simulink library "Valeo_Simulink_Library_EC"  (R2017b)
settings: Solver=ode45  StartTime=0.0  StopTime=10.0  RelTol=1e-3  EnableMultiTasking=on
undefined symbols (not defined in the file): A, B, C, Count_Max, D, InitValue, j, ke, kf, kt, L, Length, MaxIniVal, MaxVal, MinVal, NumBits1, NumBits2, P, p0, Q, R, Simulink_Library, Ts, x0
libraries: Valeo_Simulink_Library_EC x9, simulink x8, fixpt_dtprop x4
(part 3 of 3)

== system Valeo_Simulink_Library_EC/Signal_Operations/TurnOffDelay ==
  In : Inport
  Tdly : Inport  Port=2
  Te : Inport  Port=3
  CheckDly : RelationalOperator  Operator=<  OutDataTypeStr=boolean  RndMeth=Nearest  InputSameDT=on
  Check_Tdly_unsigned : fixpt_dtprop/Data Type Police Unsigned Only
      settings: SourceProductName=Simulink  SourceProductBaseCode=SL
  Check_Te_unsigned : fixpt_dtprop/Data Type Police Unsigned Only
      settings: SourceProductName=Simulink  SourceProductBaseCode=SL
  Divide : Product  Inputs=*/  OutDataTypeStr=uint32  RndMeth=Nearest  SaturateOnIntegerOverflow=on
  Inc : Constant  OutDataTypeStr=Inherit: Inherit via back propagation
  Increment : Sum  OutDataTypeStr=Inherit: Inherit via back propagation  SaturateOnIntegerOverflow=on  InputSameDT=on
  InitialCondition : Subsystem  Description=InitialCondition
  LogicalOperator : Logic  Operator=OR  AllPortsSameDT=off  OutDataTypeStr=boolean
  NewVal : UnitDelay  SampleTime=-1
  Reset : Constant  Value=0  OutDataTypeStr=Inherit: Inherit via back propagation
  ResetSwitch : Switch  Criteria=u2 ~= 0  InputSameDT=on
  StartDelay : UnitDelay  SampleTime=-1
  Out : Outport
  wires:
  LogicalOperator/1 -> Out/1
  Reset/1 -> ResetSwitch/1
  ResetSwitch/1 -> Increment/1, CheckDly/1
  Increment/1 -> NewVal/1
  CheckDly/1 -> LogicalOperator/1
  In/1 -> LogicalOperator/2, InitialCondition/1(CheckDir), StartDelay/1
  NewVal/1 -> InitialCondition/3(NewVal)
  InitialCondition/1(CalcVal) -> ResetSwitch/3
  StartDelay/1 -> ResetSwitch/2
  Divide/1 -> CheckDly/2, InitialCondition/2(Tdly)
  Te/1 -> Check_Te_unsigned/1, Divide/2
  Tdly/1 -> Check_Tdly_unsigned/1, Divide/1
  Inc/1 -> Increment/2

== system Valeo_Simulink_Library_EC/Signal_Operations/TurnOnDelay ==
  In : Inport
  Tdly : Inport  Port=2
  Te : Inport  Port=3
  CheckDly : RelationalOperator  OutDataTypeStr=boolean  RndMeth=Nearest  InputSameDT=on
  Check_Tdly_unsigned : fixpt_dtprop/Data Type Police Unsigned Only
      settings: SourceProductName=Simulink  SourceProductBaseCode=SL
  Check_Te_unsigned : fixpt_dtprop/Data Type Police Unsigned Only
      settings: SourceProductName=Simulink  SourceProductBaseCode=SL
  Divide : Product  Inputs=*/  OutDataTypeStr=uint32  SaturateOnIntegerOverflow=on
  Inc : Constant  OutDataTypeStr=Inherit: Inherit via back propagation
  Increment : Sum  OutDataTypeStr=Inherit: Inherit via back propagation  RndMeth=Simplest  SaturateOnIntegerOverflow=on  InputSameDT=on
  InitialCondition : Subsystem  Description=InitialCondition
  InitialDelayl : UnitDelay  InitialCondition=1  SampleTime=-1
  LogicalOperator : Logic  AllPortsSameDT=off  OutDataTypeStr=boolean
  NewVal : UnitDelay  SampleTime=-1
  Reset : Constant  Value=0  OutDataTypeStr=Inherit: Inherit via back propagation
  ResetSwitch : Switch  Criteria=u2 ~= 0  InputSameDT=on
  Out : Outport
  wires:
  InitialDelayl/1 -> ResetSwitch/2
  LogicalOperator/1 -> Out/1
  ResetSwitch/1 -> Increment/1, CheckDly/1
  Increment/1 -> NewVal/1
  CheckDly/1 -> LogicalOperator/1
  NewVal/1 -> InitialCondition/1(NewVal)
  In/1 -> LogicalOperator/2, InitialCondition/3(CheckDir), InitialDelayl/1
  InitialCondition/1(CalcVal) -> ResetSwitch/1
  Reset/1 -> ResetSwitch/3
  Tdly/1 -> Divide/1, Check_Tdly_unsigned/1
  Te/1 -> Divide/2, Check_Te_unsigned/1
  Divide/1 -> InitialCondition/2(Tdly), CheckDly/2
  Inc/1 -> Increment/2

== system Valeo_Simulink_Library_EC/Signal_Operations/VSL_ClarkTransformation_EC_Blk ==
  A : Inport  PortDimensions=1
  B : Inport  Port=2  PortDimensions=1
  C : Inport  Port=3  PortDimensions=1
  Calculation : Subsystem  Description=Calculations for clarke transfromation  RequirementInfo={} %GIDa_91c9902b_4297_47d8_bcc7_839692c95106
  datatype_protection : Subsystem  Description=forcing input and output to have the same data type  RequirementInfo={} %GIDa_ba0677aa_132e_4dc0_8af7_6cee4e109de7
  Alpha : Outport  RequirementInfo={} %GIDa_2f11082c_73d3_4ed4_8929_d03a8ab0ed51  PortDimensions=1
  Beta : Outport  RequirementInfo={} %GIDa_b2cc2919_a1d0_479c_944a_1162b348937b  Port=2  PortDimensions=1
  wires:
  [C] -> datatype_protection/5(C)
  [B] -> datatype_protection/4(B)
  [A] -> datatype_protection/3(A)
  Calculation/2(Beta) -> datatype_protection/2(Beta_temp)
  Calculation/1(Alpha) -> datatype_protection/1(Alpha_temp)
  datatype_protection/2(Beta) -> Beta/1
  datatype_protection/1(Alpha) -> Alpha/1
  [C] -> Calculation/3(C)
  [B] -> Calculation/2(B)
  [A] -> Calculation/1(A)
  C/1 -> [C]  "C"
  A/1 -> [A]  "A"
  B/1 -> [B]  "B"

== system Valeo_Simulink_Library_EC/Signal_Operations/VSL_InverseClarkTransformation_EC_Blk ==
  Alpha : Inport
  Beta : Inport  Port=2
  Calculations : Subsystem  Description=claclulations of Inverse clarke transform
  "DataTypeProtection " : Subsystem  Description=make sure all inputs and outputs have the same datatype
  A : Outport
  B : Outport  Port=2
  C : Outport  Port=3
  wires:
  Beta/1 -> [Beta]
  Alpha/1 -> [Alpha]
  [Beta] -> "DataTypeProtection "/5(Beta)
  [Alpha] -> "DataTypeProtection "/4(Alpha)
  [Beta] -> Calculations/2(Beta)
  [Alpha] -> Calculations/1(Alpha)
  "DataTypeProtection "/3(C) -> C/1
  "DataTypeProtection "/2(B) -> B/1
  "DataTypeProtection "/1(A) -> A/1
  Calculations/3(C) -> "DataTypeProtection "/3(C_t)
  Calculations/2(B) -> "DataTypeProtection "/2(B_t)
  Calculations/1(A) -> "DataTypeProtection "/1(A_t)

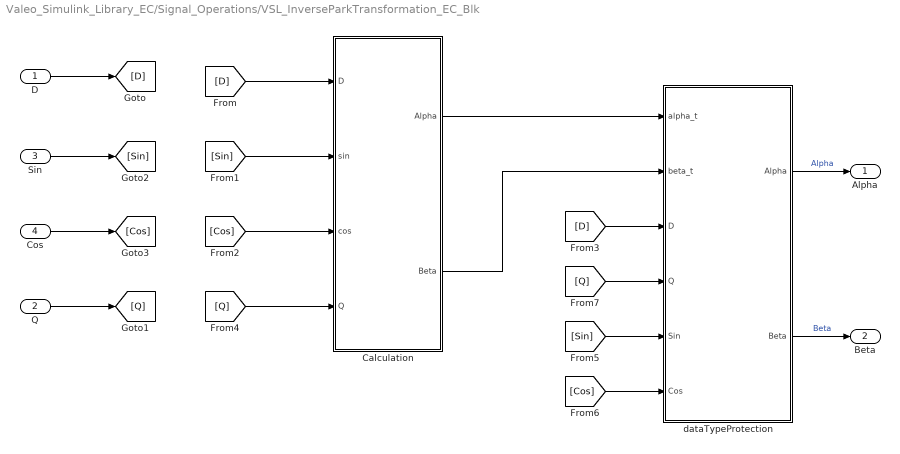
== system Valeo_Simulink_Library_EC/Signal_Operations/VSL_InverseParkTransformation_EC_Blk ==
  D : Inport
  Q : Inport  Port=2
  Sin : Inport  Port=3
  Cos : Inport  Port=4
  Calculation : Subsystem  Description=This Block is transforming dq axies with d axis aligned with Phase A into alpha-beta axises
      settings: RTWFcnNameOpts=Use subsystem name
  dataTypeProtection : Subsystem  Description=make sure inputs and outputs have the same data type
  Alpha : Outport
  Beta : Outport  Port=2
  wires:
  Calculation/1(Alpha) -> dataTypeProtection/1(alpha_t)
  Calculation/2(Beta) -> dataTypeProtection/2(beta_t)
  Q/1 -> [Q]
  D/1 -> [D]
  [D] -> Calculation/1(D)
  [Q] -> Calculation/4(Q)
  Sin/1 -> [Sin]
  Cos/1 -> [Cos]
  [Sin] -> Calculation/2(sin)
  [Cos] -> Calculation/3(cos)
  dataTypeProtection/2(Beta) -> Beta/1  "Beta"
  dataTypeProtection/1(Alpha) -> Alpha/1  "Alpha"
  [D] -> dataTypeProtection/3(D)
  [Q] -> dataTypeProtection/4(Q)
  [Sin] -> dataTypeProtection/5(Sin)
  [Cos] -> dataTypeProtection/6(Cos)

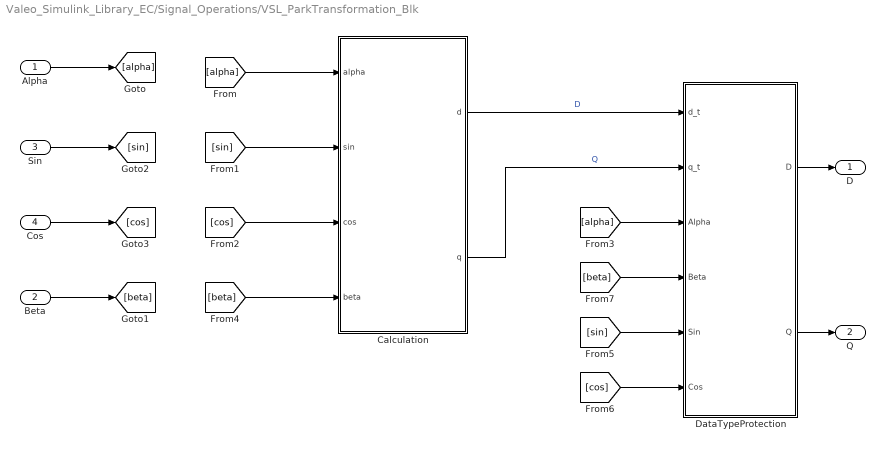
== system Valeo_Simulink_Library_EC/Signal_Operations/VSL_ParkTransformation_Blk ==
  Alpha : Inport
  Beta : Inport  Port=2
  Sin : Inport  Port=3
  Cos : Inport  Port=4
  Calculation : Subsystem  Description=This Block is transforming alpha-beta axises into dq axies with d axie aligned with Phase A
      settings: RTWSystemCode=Nonreusable function  RTWFcnNameOpts=Use subsystem name
  DataTypeProtection : Subsystem  Description=make sure all inputs and outputs have the sane data type
  D : Outport
  Q : Outport  Port=2
  wires:
  [cos] -> DataTypeProtection/6(Cos)
  [sin] -> DataTypeProtection/5(Sin)
  [beta] -> DataTypeProtection/4(Beta)
  [alpha] -> DataTypeProtection/3(Alpha)
  DataTypeProtection/2(Q) -> Q/1
  DataTypeProtection/1(D) -> D/1
  [cos] -> Calculation/3(cos)
  [sin] -> Calculation/2(sin)
  Cos/1 -> [cos]
  Sin/1 -> [sin]
  Calculation/2(q) -> DataTypeProtection/2(q_t)  "Q"
  Calculation/1(d) -> DataTypeProtection/1(d_t)  "D"
  [beta] -> Calculation/4(beta)
  [alpha] -> Calculation/1(alpha)
  Alpha/1 -> [alpha]
  Beta/1 -> [beta]

== system Valeo_Simulink_Library_EC/Utilities/EventToVar ==
  Evt : Inport
  Constant1 : Constant  Value=0  OutDataTypeStr=boolean  SampleTime=-1
  Constant2 : Constant  OutDataTypeStr=boolean  SampleTime=-1
  Function-Call Subsystem : Subsystem  Description=|  TreatAsAtomicUnit=on
      | Function-Call
      | Subsystem
  Logical Operator1 : Logic  Tag=AM,Std,Inputs,1;CMP,Operator,Inputs;  Operator=NOT  Inputs=1  AllPortsSameDT=off  OutDataTypeStr=boolean
  Relational Operator : RelationalOperator  Operator=~=  OutDataTypeStr=boolean  RndMeth=Nearest
  Switch : Switch  Criteria=u2 ~= 0
  Unit Delay1 : UnitDelay  SampleTime=-1
  Unit Delay2 : UnitDelay  SampleTime=-1
  Var : Outport
  wires:
  Logical Operator1/1 -> Relational Operator/1, Unit Delay1/1
  Switch/1 -> Var/1
  Relational Operator/1 -> Switch/2
  Constant1/1 -> Switch/3
  Constant2/1 -> Switch/1
  Unit Delay1/1 -> Relational Operator/2
  Function-Call Subsystem/1(out) -> Logical Operator1/1, Unit Delay2/1
  Unit Delay2/1 -> Function-Call Subsystem/1(in)
  Evt/1 -> Function-Call Subsystem/Trigger

== system Valeo_Simulink_Library_EC/Utilities/ScribeInfo ==

== system Valeo_Simulink_Library_EC/Plant Models/Actuators/BLDC ==
  Vs : Inport
  TL : Inport  Port=2
  BLDC motor Block : Subsystem
  inverter : Subsystem
  Te : Outport
  omega(rad/sec) : Outport  Port=2
  Position : Outport  Port=3
  i_abc : Outport  Port=4
  wires:
  BLDC motor Block/4(B_EMF) -> inverter/3(B_EMF)
  BLDC motor Block/1(Te) -> Te/1
  BLDC motor Block/3(Position) -> Position/1, inverter/1(POS)
  inverter/1("Uab, Ubc") -> BLDC motor Block/1(" Uab,Ubc")
  TL/1 -> BLDC motor Block/2(Tl)
  BLDC motor Block/5(i_abc) -> inverter/4(i_abc), i_abc/1
  Vs/1 -> inverter/2(Vs)
  BLDC motor Block/2(Omega) -> omega(rad/sec)/1  "omega(rad/sec)"

== system Valeo_Simulink_Library_EC/Signal_Operations/Debouncing_Blk/Else ==
  In : Inport
  Action Port : ActionPort
  Signal Conversion : SignalConversion  OverrideOpt=off
  Out : Outport
  wires:
  In/1 -> Signal Conversion/1
  Signal Conversion/1 -> Out/1

== system Valeo_Simulink_Library_EC/Signal_Operations/Debouncing_Blk/Turn_OFF ==
  Action Port : ActionPort
  Constant1 : Constant  Value=0  OutDataTypeStr=uint8  SampleTime=-1
  Constant3 : Constant  Value=0  OutDataTypeStr=boolean  SampleTime=-1
  Counter : Outport
  Out : Outport  Port=2
  wires:
  Constant3/1 -> Out/1
  Constant1/1 -> Counter/1

== system Valeo_Simulink_Library_EC/Signal_Operations/Debouncing_Blk/Turn_ON ==
  Action Port : ActionPort
  Constant3 : Constant  Value=0  OutDataTypeStr=uint8  SampleTime=-1
  Constant4 : Constant  OutDataTypeStr=boolean  SampleTime=-1
  Out : Outport
  Counter : Outport  Port=2
  wires:
  Constant4/1 -> Out/1
  Constant3/1 -> Counter/1

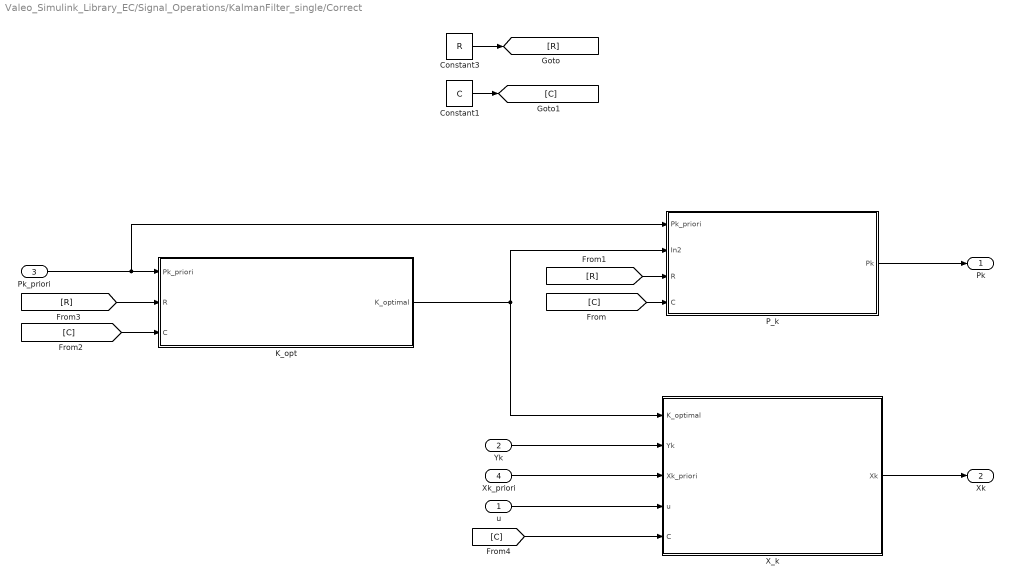
== system Valeo_Simulink_Library_EC/Signal_Operations/KalmanFilter_single/Correct ==
  u : Inport
  Yk : Inport  Port=2
  Pk_priori : Inport  Port=3
  Xk_priori : Inport  Port=4
  Constant1 : Constant  Value=C  VectorParams1D=off  OutDataTypeStr=single
  Constant3 : Constant  Value=R  VectorParams1D=off  OutDataTypeStr=single
  K_opt : Subsystem
  P_k : Subsystem
  X_k : Subsystem
  Pk : Outport  OutDataTypeStr=single  InitialOutput=0
  Xk : Outport  Port=2  OutDataTypeStr=single  InitialOutput=3
  wires:
  Pk_priori/1 -> P_k/1(Pk_priori), K_opt/1(Pk_priori)
  Constant3/1 -> [R]
  Yk/1 -> X_k/2(Yk)
  Xk_priori/1 -> X_k/3(Xk_priori)
  u/1 -> X_k/4(u)
  X_k/1(Xk) -> Xk/1
  Constant1/1 -> [C]
  [C] -> X_k/5(C)
  K_opt/1(K_optimal) -> X_k/1(K_optimal), P_k/2(In2)
  P_k/1(Pk) -> Pk/1
  [R] -> P_k/3(R)
  [C] -> P_k/4(C)
  [R] -> K_opt/2(R)
  [C] -> K_opt/3(C)

== system Valeo_Simulink_Library_EC/Signal_Operations/KalmanFilter_single/Predict ==
  u : Inport
  Pk-1 : Inport  Port=2
  Xk-1 : Inport  Port=3
  Add : Sum
  Add1 : Sum
  Constant : Constant  Value=A  VectorParams1D=off  OutDataTypeStr=single
  Constant1 : Constant  Value=Q  VectorParams1D=off  OutDataTypeStr=single
  Constant2 : Constant  Value=B  VectorParams1D=off  OutDataTypeStr=single
  Math Function : Math  Operator=transpose  SaturateOnIntegerOverflow=on
  Product : Product  Inputs=3  Multiplication=Matrix(*)
  Product1 : Product  Inputs=**  Multiplication=Matrix(*)  RndMeth=Zero
  Product2 : Product  Inputs=**  Multiplication=Matrix(*)  RndMeth=Zero
  Pk_priori : Outport  OutDataTypeStr=single
  Xk_priori : Outport  Port=2  OutDataTypeStr=single
  wires:
  Constant2/1 -> Product2/1
  Math Function/1 -> Product/3
  Constant/1 -> Product/1, Product1/1, Math Function/1
  Product/1 -> Add1/2
  Pk-1/1 -> Product/2
  Product1/1 -> Add/1
  Xk-1/1 -> Product1/2
  u/1 -> Product2/2
  Product2/1 -> Add/2
  Add1/1 -> Pk_priori/1
  Constant1/1 -> Add1/1
  Add/1 -> Xk_priori/1

== system Valeo_Simulink_Library_EC/Signal_Operations/NegHys/Hysteresis ==
  Low : Inport
  In : Inport  Port=2
  High : Inport  Port=3
  RemainderIN : Inport  Port=4
  Constant : Constant  Value=0  OutDataTypeStr=boolean
  Constant1 : Constant  OutDataTypeStr=boolean
  RelationalOperator3 : RelationalOperator  OutDataTypeStr=boolean  RndMeth=Nearest  InputSameDT=on
  RelationalOperator4 : RelationalOperator  OutDataTypeStr=boolean  RndMeth=Nearest  InputSameDT=on
  Switch : Switch  Criteria=u2 ~= 0  OutDataTypeStr=Inherit: Inherit via back propagation  InputSameDT=on
  Switch1 : Switch  Criteria=u2 ~= 0  OutDataTypeStr=Inherit: Inherit via back propagation  InputSameDT=on
  Out : Outport
  wires:
  RemainderIN/1 -> Switch1/3
  Switch/1 -> Out/1
  Switch1/1 -> Switch/3
  RelationalOperator4/1 -> Switch1/2
  Constant/1 -> Switch1/1
  RelationalOperator3/1 -> Switch/2
  Constant1/1 -> Switch/1
  Low/1 -> RelationalOperator3/1
  High/1 -> RelationalOperator4/2
  In/1 -> RelationalOperator4/1, RelationalOperator3/2

== system Valeo_Simulink_Library_EC/Signal_Operations/PosHys/Hysteresis ==
  Low : Inport
  In : Inport  Port=2
  High : Inport  Port=3
  RemainderIN : Inport  Port=4
  Constant : Constant  OutDataTypeStr=boolean
  Constant1 : Constant  Value=0  OutDataTypeStr=boolean
  RelationalOperator3 : RelationalOperator  OutDataTypeStr=boolean  RndMeth=Nearest  InputSameDT=on
  RelationalOperator4 : RelationalOperator  OutDataTypeStr=boolean  RndMeth=Nearest  InputSameDT=on
  Switch : Switch  Criteria=u2 ~= 0  OutDataTypeStr=Inherit: Inherit via back propagation  InputSameDT=on
  Switch1 : Switch  Criteria=u2 ~= 0  OutDataTypeStr=Inherit: Inherit via back propagation  InputSameDT=on
  Out : Outport
  wires:
  In/1 -> RelationalOperator3/2, RelationalOperator4/1
  High/1 -> RelationalOperator4/2
  Low/1 -> RelationalOperator3/1
  Constant1/1 -> Switch/1
  RelationalOperator3/1 -> Switch/2
  Constant/1 -> Switch1/1
  RelationalOperator4/1 -> Switch1/2
  Switch1/1 -> Switch/3
  Switch/1 -> Out/1
  RemainderIN/1 -> Switch1/3

== system Valeo_Simulink_Library_EC/Signal_Operations/SlidingAverageFiltrer/DPropagation_32Bits ==
  Ref1 : Inport
  DataProp : Inport  Port=2
  Data Type Propagation : simulink/Signal Attributes/Data Type Propagation  PropDataType=fixdt(1, 16)  IfRefDouble=double  IfRefSingle=single  IsSigned=TRUE  NumBitsBase=NumBits1  NumBitsMult=1  NumBitsAdd=0  NumBitsAllowFinal=8:32  PropScaling=2^-10  ValuesUsedBestPrec=[5 -7]  SlopeBase=Slope1  SlopeMult=1  SlopeAdd=0  BiasBase=Bias1  BiasMult=1  BiasAdd=0
      settings: SourceProductName=Simulink  SourceProductBaseCode=SL
  wires:
  Ref1/1 -> Data Type Propagation/2, Data Type Propagation/1
  DataProp/1 -> Data Type Propagation/3

== system Valeo_Simulink_Library_EC/Signal_Operations/SlidingAverageFiltrer/DPropagation_Others ==
  Ref1 : Inport
  DataProp : Inport  Port=2
  Data Type Propagation : simulink/Signal Attributes/Data Type Propagation  PropDataType=fixdt(1, 16)  IfRefDouble=double  IfRefSingle=single  IsSigned=TRUE  NumBitsBase=NumBits1+NumBits2  NumBitsMult=1  NumBitsAdd=0  NumBitsAllowFinal=8:32  PropScaling=2^-10  ValuesUsedBestPrec=[5 -7]  SlopeBase=Slope1  SlopeMult=1  SlopeAdd=0  BiasBase=Bias1  BiasMult=1  BiasAdd=0
      settings: SourceProductName=Simulink  SourceProductBaseCode=SL
  wires:
  DataProp/1 -> Data Type Propagation/3
  Ref1/1 -> Data Type Propagation/2, Data Type Propagation/1

== system Valeo_Simulink_Library_EC/Signal_Operations/SlidingAverageFiltrer/DPropagation_WindowLength ==
  Ref1 : Inport
  Ref2 : Inport  Port=2
  Prop : Inport  Port=3
  Data Type Propagation : simulink/Signal Attributes/Data Type Propagation  PropDataType=fixdt(1, 16)  IfRefDouble=double  IfRefSingle=single  IsSigned=FALSE  NumBitsBase=NumBits1  NumBitsMult=1  NumBitsAdd=0  NumBitsAllowFinal=8:32  PropScaling=2^-10  ValuesUsedBestPrec=[5 -7]  SlopeBase=Slope1  SlopeMult=1  SlopeAdd=0  BiasBase=Bias1  BiasMult=1  BiasAdd=0
      settings: SourceProductName=Simulink  SourceProductBaseCode=SL
  wires:
  Ref1/1 -> Data Type Propagation/1
  Ref2/1 -> Data Type Propagation/2
  Prop/1 -> Data Type Propagation/3

== system Valeo_Simulink_Library_EC/Signal_Operations/TurnOffDelay/InitialCondition ==
  CheckDir : Inport
  Tdly : Inport  Port=2
  NewVal : Inport  Port=3
  LogicalOperator1 : Logic  Operator=OR  AllPortsSameDT=off  OutDataTypeStr=boolean
  NewVal1 : UnitDelay  InitialCondition=1  SampleTime=-1
  Reset : Constant  Value=0  OutDataTypeStr=boolean
  Switch : Switch  Criteria=u2 ~= 0  InputSameDT=on
  CalcVal : Outport
  wires:
  NewVal/1 -> Switch/3
  Tdly/1 -> Switch/1
  NewVal1/1 -> LogicalOperator1/2
  Reset/1 -> NewVal1/1
  LogicalOperator1/1 -> Switch/2
  CheckDir/1 -> LogicalOperator1/1
  Switch/1 -> CalcVal/1

== system Valeo_Simulink_Library_EC/Signal_Operations/TurnOnDelay/InitialCondition ==
  NewVal : Inport
  Tdly : Inport  Port=2
  CheckDir : Inport  Port=3
  LogicalOperator : Logic  Operator=NOT  AllPortsSameDT=off  OutDataTypeStr=boolean
  LogicalOperator1 : Logic  Operator=OR  AllPortsSameDT=off  OutDataTypeStr=boolean
  NewVal1 : UnitDelay  SampleTime=-1
  Reset : Constant  OutDataTypeStr=boolean
  Switch : Switch  Criteria=u2 ~= 0  InputSameDT=on
  CalcVal : Outport
  wires:
  NewVal/1 -> Switch/1
  NewVal1/1 -> LogicalOperator1/2
  Reset/1 -> NewVal1/1
  LogicalOperator1/1 -> Switch/2
  Switch/1 -> CalcVal/1
  Tdly/1 -> Switch/3
  CheckDir/1 -> LogicalOperator/1
  LogicalOperator/1 -> LogicalOperator1/1

== system Valeo_Simulink_Library_EC/Signal_Operations/VSL_ClarkTransformation_EC_Blk/Calculation ==
  A : Inport
  B : Inport  Port=2
  C : Inport  Port=3
  Add : Sum  RequirementInfo={} %GIDa_afe2c577_734f_4faf_b375_0ef20aeeab01  Inputs=+++  OutDataTypeStr=Inherit: Inherit via back propagation  RndMeth=Simplest
  Add1 : Sum  RequirementInfo={} %GIDa_b8b12de4_a1c3_404a_a9d1_be098477dac5  OutDataTypeStr=Inherit: Inherit via back propagation  RndMeth=Simplest
  Const_2Over3 : Gain  Description=gain of 0.666 as 0.666  RequirementInfo={} %GIDa_120f91ab_5e07_4588_9a66_f8fa17d7ebbb  Gain=0.6667  OutDataTypeStr=Inherit: Inherit via back propagation  RndMeth=Simplest  ParamDataTypeStr=Inherit: Same as input
  Const_Neg1Over3 : Gain  Description=gain of -.333 as -.333  RequirementInfo={} %GIDa_cbff4a56_eba5_4d1b_82e9_2b912c46c30a  Gain=-.3333  OutDataTypeStr=Inherit: Inherit via back propagation  RndMeth=Simplest  ParamDataTypeStr=Inherit: Same as input
  Const_Neg1Over3_2 : Gain  Description=gain of -.333 as -.333  RequirementInfo={} %GIDa_82831831_6244_46f4_8700_983a6e4d662e  Gain=-.3333  OutDataTypeStr=Inherit: Inherit via back propagation  RndMeth=Simplest  ParamDataTypeStr=Inherit: Same as input
  Const_NegSqrt3Over3 : Gain  Description=gain of -.577 as -sqrt(3)/3  RequirementInfo={} %GIDa_a4218fb9_5262_4d86_8cc2_5cb31cf1db53  Gain=-.5773  OutDataTypeStr=Inherit: Inherit via back propagation  RndMeth=Simplest  ParamDataTypeStr=Inherit: Same as input
  Const_Sqrt3Over2 : Gain  Description=gain of .577 as sqrt(3)/3  RequirementInfo={} %GIDa_f78375a3_f7cc_4d79_b4c2_30115ac82f8c  Gain=.5773  OutDataTypeStr=Inherit: Inherit via back propagation  RndMeth=Simplest  ParamDataTypeStr=Inherit: Same as input
  Alpha : Outport
  Beta : Outport  Port=2
  wires:
  Const_Sqrt3Over2/1 -> Add1/1
  Add1/1 -> Beta/1  "Beta"
  C/1 -> Const_NegSqrt3Over3/1, Const_Neg1Over3_2/1
  A/1 -> Const_2Over3/1
  Add/1 -> Alpha/1  "Alpha"
  Const_Neg1Over3_2/1 -> Add/3
  B/1 -> Const_Neg1Over3/1, Const_Sqrt3Over2/1
  Const_Neg1Over3/1 -> Add/1
  Const_2Over3/1 -> Add/2
  Const_NegSqrt3Over3/1 -> Add1/2

== system Valeo_Simulink_Library_EC/Signal_Operations/VSL_ClarkTransformation_EC_Blk/datatype_protection ==
  Alpha_temp : Inport  PortDimensions=1
  Beta_temp : Inport  Port=2  PortDimensions=1
  A : Inport  Port=3  PortDimensions=1
  B : Inport  Port=4  PortDimensions=1
  C : Inport  Port=5  PortDimensions=1
  Data Type Duplicate : DataTypeDuplicate  RequirementInfo={} %GIDa_59c1057f_2c2c_4435_a6e2_f9e4eb9c7f02  NumInputPorts=5
  Alpha : Outport
  Beta : Outport  Port=2
  wires:
  Alpha_temp/1 -> Data Type Duplicate/1, Alpha/1
  Beta_temp/1 -> Data Type Duplicate/5, Beta/1
  C/1 -> Data Type Duplicate/4
  B/1 -> Data Type Duplicate/3
  A/1 -> Data Type Duplicate/2

== system Valeo_Simulink_Library_EC/Signal_Operations/VSL_InverseClarkTransformation_EC_Blk/Calculations ==
  Alpha : Inport
  Beta : Inport  Port=2
  Add1 : Sum  OutDataTypeStr=Inherit: Inherit via back propagation  RndMeth=Simplest
  Add2 : Sum  OutDataTypeStr=Inherit: Inherit via back propagation  RndMeth=Simplest
  Const_1Over2 : Gain  Description=-1/2  Gain=-0.5  OutDataTypeStr=Inherit: Inherit via back propagation  RndMeth=Simplest  ParamDataTypeStr=Inherit: Same as input
      settings: AttributesFormatString=%<ShowName>
  Const_NegSqrt3Over3 : Gain  Description=-Sqrt(3)/3  Gain=-.5773  OutDataTypeStr=Inherit: Inherit via back propagation  RndMeth=Simplest  ParamDataTypeStr=Inherit: Same as input
      settings: AttributesFormatString=%<ShowName>
  Const_Sqrt3Over3 : Gain  Description=Sqrt(3)/3  Gain=0.5773  OutDataTypeStr=Inherit: Inherit via back propagation  RndMeth=Simplest  ParamDataTypeStr=Inherit: Same as input
      settings: AttributesFormatString=%<ShowName>
  Signal Conversion : SignalConversion  OverrideOpt=off
  A : Outport
  B : Outport  Port=2
  C : Outport  Port=3
  wires:
  Alpha/1 -> Const_1Over2/1, Signal Conversion/1
  Beta/1 -> Const_NegSqrt3Over3/1, Const_Sqrt3Over3/1
  Add1/1 -> B/1  "B"
  Const_1Over2/1 -> Add2/2, Add1/2
  Const_Sqrt3Over3/1 -> Add1/1
  Signal Conversion/1 -> A/1  "A"
  Add2/1 -> C/1  "C"
  Const_NegSqrt3Over3/1 -> Add2/1

== system Valeo_Simulink_Library_EC/Signal_Operations/VSL_InverseClarkTransformation_EC_Blk/DataTypeProtection  ==
  A_t : Inport
  B_t : Inport  Port=2
  C_t : Inport  Port=3
  Alpha : Inport  Port=4
  Beta : Inport  Port=5
  Data Type Duplicate : DataTypeDuplicate  NumInputPorts=5
  A : Outport
  B : Outport  Port=2
  C : Outport  Port=3
  wires:
  Alpha/1 -> Data Type Duplicate/4
  Beta/1 -> Data Type Duplicate/5
  C_t/1 -> Data Type Duplicate/3, C/1
  A_t/1 -> Data Type Duplicate/1, A/1
  B_t/1 -> Data Type Duplicate/2, B/1

== system Valeo_Simulink_Library_EC/Signal_Operations/VSL_InverseParkTransformation_EC_Blk/Calculation ==
  D : Inport
  sin : Inport  Port=2
  cos : Inport  Port=3
  Q : Inport  Port=4
  Add : Sum  Inputs=-+
  Add1 : Sum
  Multiply{,1..3} (4 alike) : Product  OutDataTypeStr=Inherit: Inherit via back propagation
  Alpha : Outport
  Beta : Outport  Port=2
  wires:
  Add/1 -> Alpha/1
  [q] -> Multiply1/1
  [q] -> Multiply3/1
  Multiply3/1 -> Add1/2
  Multiply2/1 -> Add/2
  cos/1 -> Multiply3/2, Multiply2/2
  Multiply/1 -> Add1/1
  sin/1 -> Multiply/2, Multiply1/2
  Multiply1/1 -> Add/1
  [d] -> Multiply2/1
  D/1 -> [d]
  Q/1 -> [q]
  [d] -> Multiply/1
  Add1/1 -> Beta/1

== system Valeo_Simulink_Library_EC/Signal_Operations/VSL_InverseParkTransformation_EC_Blk/dataTypeProtection ==
  alpha_t : Inport
  beta_t : Inport  Port=2
  D : Inport  Port=3
  Q : Inport  Port=4
  Sin : Inport  Port=5
  Cos : Inport  Port=6
  Data Type Duplicate : DataTypeDuplicate
  Data Type Duplicate1 : DataTypeDuplicate  NumInputPorts=4
  Alpha : Outport
  Beta : Outport  Port=2
  wires:
  alpha_t/1 -> Alpha/1, Data Type Duplicate1/1
  Sin/1 -> Data Type Duplicate/1
  Cos/1 -> Data Type Duplicate/2
  beta_t/1 -> Data Type Duplicate1/4, Beta/1
  Q/1 -> Data Type Duplicate1/3
  D/1 -> Data Type Duplicate1/2

== system Valeo_Simulink_Library_EC/Signal_Operations/VSL_ParkTransformation_Blk/Calculation ==
  alpha : Inport
  sin : Inport  Port=2
  cos : Inport  Port=3
  beta : Inport  Port=4
  Add : Sum  OutDataTypeStr=Inherit: Inherit via back propagation  RndMeth=Simplest
  Add1 : Sum  Inputs=-+  OutDataTypeStr=Inherit: Inherit via back propagation  RndMeth=Simplest
  Multiply{,1..3} (4 alike) : Product  OutDataTypeStr=Inherit: Inherit via back propagation  RndMeth=Simplest
  d : Outport
  q : Outport  Port=2
  wires:
  [beta] -> Multiply1/1
  Multiply2/1 -> Add/2
  Multiply1/1 -> Add/1
  Multiply3/1 -> Add1/2
  Multiply/1 -> Add1/1
  Add1/1 -> q/1
  Add/1 -> d/1
  [alpha] -> Multiply/1
  beta/1 -> [beta]
  alpha/1 -> [alpha]
  [alpha] -> Multiply2/1
  sin/1 -> Multiply1/2, Multiply/2
  [beta] -> Multiply3/1
  cos/1 -> Multiply3/2, Multiply2/2

== system Valeo_Simulink_Library_EC/Signal_Operations/VSL_ParkTransformation_Blk/DataTypeProtection ==
  d_t : Inport
  q_t : Inport  Port=2
  Alpha : Inport  Port=3
  Beta : Inport  Port=4
  Sin : Inport  Port=5
  Cos : Inport  Port=6
  Data Type Duplicate : DataTypeDuplicate  NumInputPorts=4
  Data Type Duplicate1 : DataTypeDuplicate
  D : Outport
  Q : Outport  Port=2
  wires:
  Cos/1 -> Data Type Duplicate1/2
  Sin/1 -> Data Type Duplicate1/1
  d_t/1 -> D/1, Data Type Duplicate/1
  q_t/1 -> Q/1, Data Type Duplicate/4
  Beta/1 -> Data Type Duplicate/3
  Alpha/1 -> Data Type Duplicate/2

== system Valeo_Simulink_Library_EC/Utilities/EventToVar/Function-Call Subsystem ==
  in : Inport  Tag=AM,In,0,1,Name,C;CMP,Port,PortWidth,SampleTime;
  function : TriggerPort  TriggerType=function-call  VariantControl=(inherit)  StatesWhenEnabling=reset
      settings: AttributesFormatString=%<StatesWhenEnabling>
  Logical Operator1 : Logic  Tag=AM,Std,Inputs,1;CMP,Operator,Inputs;  Operator=NOT  Inputs=1  AllPortsSameDT=off  OutDataTypeStr=boolean
  out : Outport  Tag=AM,Out,1,0,Name,NC;CMP,Port,OutputWhenDisabled,InitialOutput;  InitialOutput=1
      settings: AttributesFormatString=%<OutputWhenDisabled>
  wires:
  in/1 -> Logical Operator1/1
  Logical Operator1/1 -> out/1

== system Valeo_Simulink_Library_EC/Plant Models/Actuators/BLDC/BLDC motor Block ==
  " Uab,Ubc" : Inport
  Tl : Inport  Port=2
  Add : Sum  Inputs=+-
  Demux : Demux  Outputs=5
  Electromagnetic_Torque : Subsystem
  Gain : Gain  Gain=ke/2
  Mux : Mux  Inputs=2
  Mux1 : Mux  Inputs=3
  PhaseCurrent_speed_position : StateSpace  A=[-R/L 0 0 0;0 -R/L 0 0;0 0 -kf/j 0;0 0 1 0]  B=[2/(3*L) 1/(3*L) 0;-1/(3*L) 1/(3*L) 0;0 0 1/j;0 0 0]  C=[1 0 0 0;0 1 0 0;-1 -1 0 0;0 0 1 0;0 0 0 1]  D=zeros(5,3)  InitialCondition=x0
  Product : Product
  Trapz_f : Subsystem
  Te : Outport
  Omega : Outport  Port=2
  Position : Outport  Port=3
  B_EMF : Outport  Port=4
  i_abc : Outport  Port=5
  wires:
  Demux/5 -> Trapz_f/1(Theta_m)
  Mux1/1 -> i_abc/1, Electromagnetic_Torque/2(i_abc)  "i_abc"
  Demux/1 -> Mux1/1
  Tl/1 -> Add/2
  Demux/2 -> Mux1/2
  Trapz_f/2(f_abc) -> Product/2, Electromagnetic_Torque/1(f_abc)
  Demux/3 -> Mux1/3
  Product/1 -> Gain/1
  Mux/1 -> PhaseCurrent_speed_position/1
  Demux/4 -> Omega/1, Product/1  "omega"
  " Uab,Ubc"/1 -> Mux/1
  PhaseCurrent_speed_position/1 -> Demux/1
  Trapz_f/1(Position) -> Position/1
  Electromagnetic_Torque/1(Te) -> Te/1, Add/1  "Te"
  Add/1 -> Mux/2
  Gain/1 -> B_EMF/1

== system Valeo_Simulink_Library_EC/Plant Models/Actuators/BLDC/inverter ==
  POS : Inport
  Vs : Inport  Port=2
  B_EMF : Inport  Port=3
  i_abc : Inport  Port=4
  MATLAB Function : MATLAB Function  TreatAsAtomicUnit=on
  "Uab, Ubc" : Outport
  wires:
  POS/1 -> MATLAB Function/1(POS)
  Vs/1 -> MATLAB Function/2(Vs)
  B_EMF/1 -> MATLAB Function/3(e_abc)
  i_abc/1 -> MATLAB Function/4(i_abc)
  MATLAB Function/1(U) -> "Uab, Ubc"/1

== system Valeo_Simulink_Library_EC/Signal_Operations/KalmanFilter_single/Correct/K_opt ==
  Pk_priori : Inport
  R : Inport  Port=2
  C : Inport  Port=3
  Add : Sum
  Math Function : Math  Operator=transpose  SaturateOnIntegerOverflow=on
  Matrix Divide : Product  Inputs=/  Multiplication=Matrix(*)
  Product : Product  Inputs=3  Multiplication=Matrix(*)
  Product2 : Product  Inputs=3  Multiplication=Matrix(*)
  K_optimal : Outport
  wires:
  Pk_priori/1 -> Product/1, Product2/2
  C/1 -> Product2/1, Math Function/1
  Math Function/1 -> Product/2, Product2/3
  R/1 -> Add/2
  Matrix Divide/1 -> Product/3
  Product2/1 -> Add/1
  Add/1 -> Matrix Divide/1
  Product/1 -> K_optimal/1  "K_optimal"

== system Valeo_Simulink_Library_EC/Signal_Operations/KalmanFilter_single/Correct/P_k ==
  Pk_priori : Inport
  In2 : Inport  Port=2
  R : Inport  Port=3
  C : Inport  Port=4
  Add1 : Sum
  Add4 : Sum  Inputs=+-
  Math Function1 : Math  Operator=transpose  SaturateOnIntegerOverflow=on
  Math Function2 : Math  Operator=transpose  SaturateOnIntegerOverflow=on
  Product4 : Product  Multiplication=Matrix(*)
  Product6 : Product  Inputs=3  Multiplication=Matrix(*)
  Product7 : Product  Inputs=3  Multiplication=Matrix(*)
  Var_ident_mat : Constant  Value=eye(length(A))  VectorParams1D=off  OutDataTypeStr=single
  Pk : Outport
  wires:
  C/1 -> Product4/2
  Add1/1 -> Pk/1
  Math Function2/1 -> Product7/3
  Product4/1 -> Add4/2
  In2/1 -> Math Function2/1, Product7/1, Product4/1
  Product7/1 -> Add1/2
  R/1 -> Product7/2
  Math Function1/1 -> Product6/3
  Add4/1 -> Product6/1, Math Function1/1
  Var_ident_mat/1 -> Add4/1
  Pk_priori/1 -> Product6/2
  Product6/1 -> Add1/1

== system Valeo_Simulink_Library_EC/Signal_Operations/KalmanFilter_single/Correct/X_k ==
  K_optimal : Inport
  Yk : Inport  Port=2
  Xk_priori : Inport  Port=3
  u : Inport  Port=4
  C : Inport  Port=5
  Add2 : Sum  Inputs=+--
  Add3 : Sum
  Constant2 : Constant  Value=D  VectorParams1D=off  OutDataTypeStr=single
  Product1 : Product  Multiplication=Matrix(*)
  Product3 : Product  Multiplication=Matrix(*)
  Product5 : Product  Multiplication=Matrix(*)
  Xk : Outport  OutDataTypeStr=single  InitialOutput=3
  wires:
  Product1/1 -> Add2/2
  Add3/1 -> Xk/1
  Xk_priori/1 -> Product1/2, Add3/2
  K_optimal/1 -> Product3/1
  u/1 -> Product5/2
  Yk/1 -> Add2/1
  Product5/1 -> Add2/3
  Product3/1 -> Add3/1
  Constant2/1 -> Product5/1
  Add2/1 -> Product3/2
  C/1 -> Product1/1

== system Valeo_Simulink_Library_EC/Plant Models/Actuators/BLDC/BLDC motor Block/Electromagnetic_Torque ==
  f_abc : Inport
  i_abc : Inport  Port=2
  Dot Product : DotProduct  InputSameDT=on  OutDataTypeStr=Inherit: Inherit via internal rule
  Gain : Gain  Gain=kt/2
  Te : Outport
  wires:
  f_abc/1 -> Dot Product/1
  i_abc/1 -> Dot Product/2
  Dot Product/1 -> Gain/1
  Gain/1 -> Te/1

== system Valeo_Simulink_Library_EC/Plant Models/Actuators/BLDC/BLDC motor Block/Trapz_f ==
  note: sinusoidal BEMF
  note: Instead of Position range: 0-5, output can be mapped to HALL sensor readings,
      | then inverter logic must be changed accordingly!
  Theta_m : Inport
  1-D Lookup Table : Lookup_n-D  NumberOfTableDimensions=1  BreakpointsForDimension1=0:pi/3:2*pi  Table=[1 1 1 -1 -1 -1 1]  RndMeth=Simplest  InputSameDT=on
  1-D Lookup Table1 : Lookup_n-D  NumberOfTableDimensions=1  BreakpointsForDimension1=0:pi/3:2*pi  Table=[-1 -1 1 1 1 -1 -1]  RndMeth=Simplest  InputSameDT=on
  1-D Lookup Table2 : Lookup_n-D  NumberOfTableDimensions=1  BreakpointsForDimension1=0:pi/3:2*pi  Table=[1 -1 -1 -1 1 1 1]  RndMeth=Simplest  InputSameDT=on
  1-D Lookup Table3 : Lookup_n-D  NumberOfTableDimensions=1  BreakpointsForDimension1=[0 1.047 pi/3 2.0942 2*pi/3 3.1414 pi 4.1886 4*pi/3 5.2358 5*pi/3 6.283 ]  Table=[0 0 1 1 2 2 3 3 4 4 5 5]  TableDataTypeStr=uint8  ExtrapMethod=Clip  OutDataTypeStr=uint8  RndMeth=Simplest  InputSameDT=on
  Fcn : Fcn  Expr=rem(u,2*pi)
  Gain : Gain  Gain=P/2
  Manual Switch : ManualSwitch  CurrentSetting=0
  Mux : Mux  Inputs=3
  Mux1 : Mux  Inputs=3
  Scope : Scope
  Sine Wave : Sin  TimeSource=Use external signal  SampleTime=0
  Sine Wave1 : Sin  TimeSource=Use external signal  Phase=-2*pi/3  SampleTime=0
  Sine Wave2 : Sin  TimeSource=Use external signal  Phase=-4*pi/3  SampleTime=0
  Position : Outport
  f_abc : Outport  Port=2
  wires:
  Theta_m/1 -> Gain/1
  Gain/1 -> Fcn/1
  1-D Lookup Table/1 -> Mux/1
  1-D Lookup Table1/1 -> Mux/2
  1-D Lookup Table2/1 -> Mux/3
  Mux/1 -> Manual Switch/2  "trapz"
  Fcn/1 -> 1-D Lookup Table3/1, 1-D Lookup Table2/1, 1-D Lookup Table/1, Sine Wave/1, Sine Wave1/1, Sine Wave2/1, 1-D Lookup Table1/1  "Theta_e"
  1-D Lookup Table3/1 -> Position/1
  Sine Wave2/1 -> Mux1/3
  Sine Wave1/1 -> Mux1/2
  Sine Wave/1 -> Mux1/1
  Mux1/1 -> Manual Switch/1  "sin"
  Manual Switch/1 -> Scope/1, f_abc/1

== matlab function Valeo_Simulink_Library_EC/Plant Models/Actuators/BLDC/inverter/MATLAB Function ==
  data: POS input; Vs input; e_abc input; U output; i_abc input
function U = inverter(POS,Vs,e_abc,i_abc)
%U: [Vab-Eab;Vbc-Ebc]
ebs=0.00000001;% comparing to zero destabilize the solver

if (POS==0) && (i_abc(3)>ebs) 
U= [Vs-e_abc(1)+e_abc(2);-e_abc(2)+e_abc(3)];
elseif  (POS==0) && (i_abc(3)<=ebs)
U= [Vs-e_abc(1)+e_abc(2);0.5*(-Vs+e_abc(1)-e_abc(2))];

elseif (POS==1) && (i_abc(2)<ebs)
U= [-e_abc(1)+e_abc(2);Vs-e_abc(2)+e_abc(3)];
elseif  (POS==1) && (i_abc(2)>=ebs)
U= [0.5*(Vs-e_abc(1)+e_abc(3));0.5*(Vs-e_abc(1)+e_abc(3))];

elseif (POS==2) && (i_abc(1)>ebs)
U= [-Vs-e_abc(1)+e_abc(2);Vs-e_abc(2)+e_abc(3)];
elseif  (POS==2) && (i_abc(1)<=ebs)
U= [0.5*(-Vs+e_abc(2)-e_abc(3));Vs-e_abc(2)+e_abc(3)];

elseif (POS==3)&& (i_abc(3)<ebs)
U= [-Vs-e_abc(1)+e_abc(2);-e_abc(2)+e_abc(3)];
elseif  (POS==3) && (i_abc(3)>=ebs)
U= [-Vs-e_abc(1)+e_abc(2);0.5*(Vs+e_abc(1)-e_abc(2))];

elseif (POS==4) && (i_abc(2)>ebs)
U= [-e_abc(1)+e_abc(2);-Vs-e_abc(2)+e_abc(3)];
elseif   (POS==4) && (i_abc(2)<=ebs)
U= [0.5*(-Vs-e_abc(1)+e_abc(3));0.5*(-Vs-e_abc(1)+e_abc(3))];

elseif (POS==5) && (i_abc(1)<ebs)
U= [Vs-e_abc(1)+e_abc(2);-Vs-e_abc(2)+e_abc(3)];
elseif   (POS==5) && (i_abc(1)>=ebs)
U= [0.5*(Vs+e_abc(2)-e_abc(3));-Vs-e_abc(2)+e_abc(3)];

 else
 U=[0.0;0.0]; % has no contribution to calculation , but it must be included as a work around to an error of 
end
